simulink model "heat_exchanger_conditioning"  (R2020a)
settings: Solver=VariableStepAuto  StartTime=0.0  StopTime=1.0  RelTol=1e-3
settings Model: Creator=Mertcan  LastModifiedBy=Mertcan

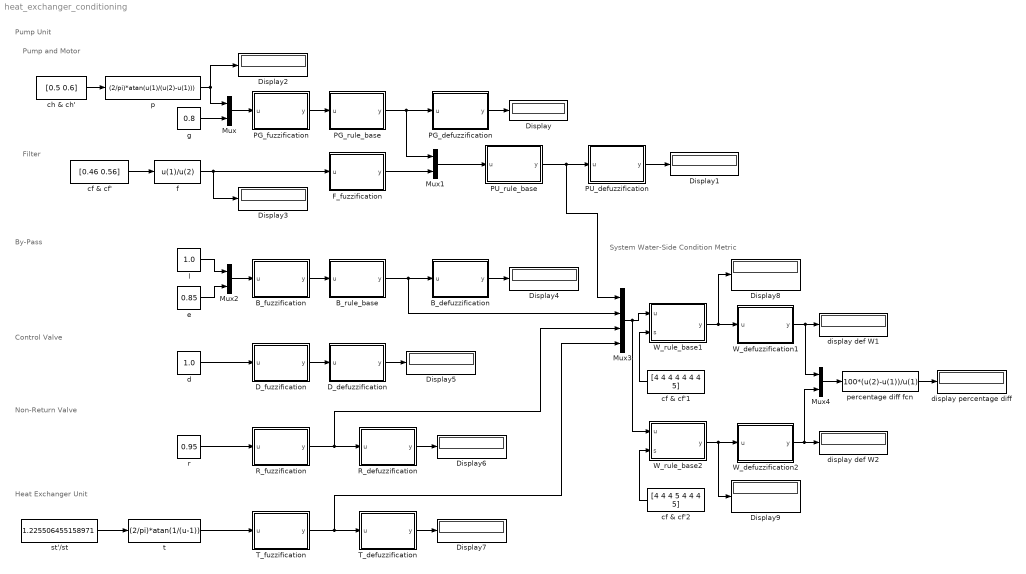
== system heat_exchanger_conditioning ==
  note: System Water-Side Condition Metric
  note: Filter
  note: Pump and Motor
  note: Heat Exchanger Unit
  note: Non-Return Valve
  note: Control Valve
  note: By-Pass
  note: Pump Unit
  B_defuzzification : MATLAB Function  TreatAsAtomicUnit=on
  B_fuzzification : MATLAB Function  TreatAsAtomicUnit=on
  B_rule_base : MATLAB Function  TreatAsAtomicUnit=on
  D_defuzzification : MATLAB Function  TreatAsAtomicUnit=on
  D_fuzzification : MATLAB Function  TreatAsAtomicUnit=on
  Display{,1..9} (10 alike) : Display
  F_fuzzification : MATLAB Function  TreatAsAtomicUnit=on
  Mux{,1..2,4} (4 alike) : Mux  Inputs=2
  Mux3 : Mux
  PG_defuzzification : MATLAB Function  TreatAsAtomicUnit=on
  PG_fuzzification : MATLAB Function  TreatAsAtomicUnit=on
  PG_rule_base : MATLAB Function  TreatAsAtomicUnit=on
  PU_defuzzification : MATLAB Function  TreatAsAtomicUnit=on
  PU_rule_base : MATLAB Function  TreatAsAtomicUnit=on
  R_defuzzification : MATLAB Function  TreatAsAtomicUnit=on
  R_fuzzification : MATLAB Function  TreatAsAtomicUnit=on
  T_defuzzification : MATLAB Function  TreatAsAtomicUnit=on
  T_fuzzification : MATLAB Function  TreatAsAtomicUnit=on
  W_defuzzification1 : MATLAB Function  TreatAsAtomicUnit=on
  W_defuzzification2 : MATLAB Function  TreatAsAtomicUnit=on
  W_rule_base1 : MATLAB Function  TreatAsAtomicUnit=on
  W_rule_base2 : MATLAB Function  TreatAsAtomicUnit=on
  cf & cf' : Constant  Value=[0.46 0.56]
  cf & cf'1 : Constant  Value=[4 4 4 4 4 4 4 5]
  cf & cf'2 : Constant  Value=[4 4 4 5 4 4 4 5]
  ch & ch' : Constant  Value=[0.5 0.6]
  d : Constant  Value=1.0
  display def W1 : Display
  display def W2 : Display
  display percentage diff : Display
  e : Constant  Value=0.85
  f : Fcn  Expr=u(1)/u(2)
  g : Constant  Value=0.8
  l : Constant  Value=1.0
  p : Fcn  Expr=(2/pi)*atan(u(1)/(u(2)-u(1)))
  percentage diff fcn : Fcn  Expr=100*(u(2)-u(1))/u(1)
  r : Constant  Value=0.95
  st'/st : Constant  Value=1.225506455158971
  t : Fcn  Expr=(2/pi)*atan(1/(u-1))
  wires:
  p/1 -> Display2/1, Mux/1
  g/1 -> Mux/2
  Mux/1 -> PG_fuzzification/1(u)
  f/1 -> Display3/1, F_fuzzification/1(u)
  PG_fuzzification/1(y) -> PG_rule_base/1(u)
  PU_defuzzification/1(y) -> Display1/1
  ch & ch'/1 -> p/1
  cf & cf'/1 -> f/1
  e/1 -> Mux2/2
  l/1 -> Mux2/1
  Mux2/1 -> B_fuzzification/1(u)
  B_fuzzification/1(y) -> B_rule_base/1(u)
  d/1 -> D_fuzzification/1(u)
  r/1 -> R_fuzzification/1(u)
  t/1 -> T_fuzzification/1(u)
  st'/st/1 -> t/1
  PG_rule_base/1(y) -> PG_defuzzification/1(u), Mux1/1
  PG_defuzzification/1(y) -> Display/1
  Mux1/1 -> PU_rule_base/1(u)
  PU_rule_base/1(y) -> Mux3/1, PU_defuzzification/1(u)
  F_fuzzification/1(y) -> Mux1/2
  B_rule_base/1(y) -> Mux3/2, B_defuzzification/1(u)
  B_defuzzification/1(y) -> Display4/1
  D_defuzzification/1(y) -> Display5/1
  D_fuzzification/1(y) -> D_defuzzification/1(u)
  R_defuzzification/1(y) -> Display6/1
  R_fuzzification/1(y) -> Mux3/3, R_defuzzification/1(u)
  T_fuzzification/1(y) -> Mux3/4, T_defuzzification/1(u)
  T_defuzzification/1(y) -> Display7/1
  Mux3/1 -> W_rule_base2/1(u), W_rule_base1/1(u)
  cf & cf'1/1 -> W_rule_base1/2(s)
  cf & cf'2/1 -> W_rule_base2/2(s)
  W_rule_base1/1(y) -> W_defuzzification1/1(u), Display8/1
  W_rule_base2/1(y) -> W_defuzzification2/1(u), Display9/1
  W_defuzzification1/1(y) -> Mux4/1, display def W1/1
  W_defuzzification2/1(y) -> Mux4/2, display def W2/1
  Mux4/1 -> percentage diff fcn/1
  percentage diff fcn/1 -> display percentage diff/1

== matlab function heat_exchanger_conditioning/T_fuzzification ==
  data: u input; y output
function y = fcn(u)

% Heat Exchanger Unit
t = u; % pump condition

T = epud(t);

y = T;

function mu = epud(x)
    mu = zeros(1,5);
    if x < 0
        mu(1) = 1+4*x;
    elseif x < 0.25
        mu(1) = 1-4*x;
        mu(2) = 4*x;
    elseif x < 0.5
        mu(2) = 2*(1-2*x);
        mu(3) = 4*x-1;
    elseif x < 0.75
        mu(3) = 3-4*x;
        mu(4) = 2*(2*x-1);
    elseif x < 1
        mu(4) = 4*(1-x);
        mu(5) = 4*x-3;
    else
        mu(5) = 5-4*x;
    end
end

end

== matlab function heat_exchanger_conditioning/W_rule_base1 ==
  data: u input; y output; s input
function y = fcn(u,s)

% System Water-Side Condition Metric

% Pump Unit
PU = u(1,1:5);

% By-Pass
B = u(1,6:10);

% Control Valve
% D: reduced without loss

% Non-Return Valve
R = u(1,11:15);

% Heat Exchanger Unit
T = u(1,16:20);

firingPU = find(PU > 0);
firingB = find(B > 0);
firingR = find(R > 0);
firingT = find(T > 0);

outPU = zeros(1,2);
outPU(1) = PU(firingPU(1));
outPU(2) = PU(firingPU(2));

outB = zeros(1,2);
outB(1) = B(firingB(1));
outB(2) = B(firingB(2));

outR = zeros(1,2);
outR(1) = R(firingR(1));
outR(2) = R(firingR(2));

outT = zeros(1,2);
outT(1) = T(firingT(1));
outT(2) = T(firingT(2));

W = ruleW(outPU,outB,outR,outT,s);

y = W;

function W = ruleW(outPU,outB,outR,outT,subscript)
    
    maxPU = max(outPU);
    
    R4 = zeros(1,8);
    R5 = zeros(1,8);
    
    if subscript(1) == 4
        R4(1) = min([maxPU,outB(1),outR(1),outT(1)]);
    elseif subscript(1) == 5
        R5(1) = min([maxPU,outB(1),outR(1),outT(1)]);
    end
    if subscript(2) == 4
        R4(2) = min([maxPU,outB(1),outR(1),outT(2)]);
    elseif subscript(2) == 5
        R5(2) = min([maxPU,outB(1),outR(1),outT(2)]);
    end
    if subscript(3) == 4
        R4(3) = min([maxPU,outB(1),outR(2),outT(1)]);
    elseif subscript(3) == 5
        R5(3) = min([maxPU,outB(1),outR(2),outT(1)]);
    end
    if subscript(4) == 4
        R4(4) = min([maxPU,outB(1),outR(2),outT(2)]);
    elseif subscript(4) == 5
        R5(4) = min([maxPU,outB(1),outR(2),outT(2)]);
    end
    if subscript(5) == 4
        R4(5) = min([maxPU,outB(2),outR(1),outT(1)]);
    elseif subscript(5) == 5
        R5(5) = min([maxPU,outB(2),outR(1),outT(1)]);
    end
    if subscript(6) == 4
        R4(6) = min([maxPU,outB(2),outR(1),outT(2)]);
    elseif subscript(6) == 5
        R5(6) = min([maxPU,outB(2),outR(1),outT(2)]);
    end
    if subscript(7) == 4
        R4(7) = min([maxPU,outB(2),outR(2),outT(1)]);
    elseif subscript(7) == 5
        R5(7) = min([maxPU,outB(2),outR(2),outT(1)]);
    end
    if subscript(8) == 4
        R4(8) = min([maxPU,outB(2),outR(2),outT(2)]);
    elseif subscript(8) == 5
        R5(8) = min([maxPU,outB(2),outR(2),outT(2)]);
    end
    
	W = [max(R4),max(R5)];    
end


end

== matlab function heat_exchanger_conditioning/W_rule_base2 ==
  data: u input; y output; s input
function y = fcn(u,s)

% System Water-Side Condition Metric

% Pump Unit
PU = u(1,1:5);

% By-Pass
B = u(1,6:10);

% Control Valve
% D: reduced without loss

% Non-Return Valve
R = u(1,11:15);

% Heat Exchanger Unit
T = u(1,16:20);

firingPU = find(PU > 0);
firingB = find(B > 0);
firingR = find(R > 0);
firingT = find(T > 0);

outPU = zeros(1,2);
outPU(1) = PU(firingPU(1));
outPU(2) = PU(firingPU(2));

outB = zeros(1,2);
outB(1) = B(firingB(1));
outB(2) = B(firingB(2));

outR = zeros(1,2);
outR(1) = R(firingR(1));
outR(2) = R(firingR(2));

outT = zeros(1,2);
outT(1) = T(firingT(1));
outT(2) = T(firingT(2));

W = ruleW(outPU,outB,outR,outT,s);

y = W;

function W = ruleW(outPU,outB,outR,outT,subscript)
    
    maxPU = max(outPU);
    
    R4 = zeros(1,8);
    R5 = zeros(1,8);
    
    if subscript(1) == 4
        R4(1) = min([maxPU,outB(1),outR(1),outT(1)]);
    elseif subscript(1) == 5
        R5(1) = min([maxPU,outB(1),outR(1),outT(1)]);
    end
    if subscript(2) == 4
        R4(2) = min([maxPU,outB(1),outR(1),outT(2)]);
    elseif subscript(2) == 5
        R5(2) = min([maxPU,outB(1),outR(1),outT(2)]);
    end
    if subscript(3) == 4
        R4(3) = min([maxPU,outB(1),outR(2),outT(1)]);
    elseif subscript(3) == 5
        R5(3) = min([maxPU,outB(1),outR(2),outT(1)]);
    end
    if subscript(4) == 4
        R4(4) = min([maxPU,outB(1),outR(2),outT(2)]);
    elseif subscript(4) == 5
        R5(4) = min([maxPU,outB(1),outR(2),outT(2)]);
    end
    if subscript(5) == 4
        R4(5) = min([maxPU,outB(2),outR(1),outT(1)]);
    elseif subscript(5) == 5
        R5(5) = min([maxPU,outB(2),outR(1),outT(1)]);
    end
    if subscript(6) == 4
        R4(6) = min([maxPU,outB(2),outR(1),outT(2)]);
    elseif subscript(6) == 5
        R5(6) = min([maxPU,outB(2),outR(1),outT(2)]);
    end
    if subscript(7) == 4
        R4(7) = min([maxPU,outB(2),outR(2),outT(1)]);
    elseif subscript(7) == 5
        R5(7) = min([maxPU,outB(2),outR(2),outT(1)]);
    end
    if subscript(8) == 4
        R4(8) = min([maxPU,outB(2),outR(2),outT(2)]);
    elseif subscript(8) == 5
        R5(8) = min([maxPU,outB(2),outR(2),outT(2)]);
    end
    
	W = [max(R4),max(R5)];    
end


end

== matlab function heat_exchanger_conditioning/W_defuzzification1 ==
  data: u input; y output
function y = fcn(u)

W = zeros(1,5);
W(4) = u(1);
W(5) = u(2);

defW = defuzzify(W);

y = defW;

function out = defuzzify(R)

    out = (R(1)*0 + R(2)*0.25 + R(3)*0.5 + R(4)*0.75 + R(5)*1)/(sum(R));

end

end

== matlab function heat_exchanger_conditioning/W_defuzzification2 ==
  data: u input; y output
function y = fcn(u)

W = zeros(1,5);
W(4) = u(1);
W(5) = u(2);

defW = defuzzify(W);

y = defW;

function out = defuzzify(R)

    out = (R(1)*0 + R(2)*0.25 + R(3)*0.5 + R(4)*0.75 + R(5)*1)/(sum(R));

end

end

== matlab function heat_exchanger_conditioning/PG_fuzzification ==
  data: u input; y output
function y = fcn(u)

% Pump and Motor
p = u(1); % pump condition
g = u(2); % assumed pump-gland condition

% Pump and Filter Condition
P = epud(p); % filter condition
G = epud(g); % gland condition

y = [P;G];

function mu = epud(x)
    mu = zeros(1,5);
    if x < 0
        mu(1) = 1+4*x;
    elseif x < 0.25
        mu(1) = 1-4*x;
        mu(2) = 4*x;
    elseif x < 0.5
        mu(2) = 2*(1-2*x);
        mu(3) = 4*x-1;
    elseif x < 0.75
        mu(3) = 3-4*x;
        mu(4) = 2*(2*x-1);
    elseif x < 1
        mu(4) = 4*(1-x);
        mu(5) = 4*x-3;
    else
        mu(5) = 5-4*x;
    end
end

end

== matlab function heat_exchanger_conditioning/B_fuzzification ==
  data: u input; y output
function y = fcn(u)

% By-Pass
l = u(1); % observed valve gland seal condition

L = epud(l);

e = u(2); % operational ease condition

E = epud_inv(e);

y = [L,E];

function mu = epud(x)
    mu = zeros(1,5);
    if x < 0
        mu(1) = 1+4*x;
    elseif x < 0.25
        mu(1) = 1-4*x;
        mu(2) = 4*x;
    elseif x < 0.5
        mu(2) = 2*(1-2*x);
        mu(3) = 4*x-1;
    elseif x < 0.75
        mu(3) = 3-4*x;
        mu(4) = 2*(2*x-1);
    elseif x < 1
        mu(4) = 4*(1-x);
        mu(5) = 4*x-3;
    else
        mu(5) = 5-4*x;
    end
end

function mu = epud_inv(x)
    mu = zeros(1,5);
    if x < 0
        mu(5) = 1+4*x;
    elseif x < 0.25
        mu(5) = 1-4*x;
        mu(4) = 4*x;
    elseif x < 0.5
        mu(4) = 2*(1-2*x);
        mu(3) = 4*x-1;
    elseif x < 0.75
        mu(3) = 3-4*x;
        mu(2) = 2*(2*x-1);
    elseif x < 1
        mu(2) = 4*(1-x);
        mu(1) = 4*x-3;
    else
        mu(1) = 5-4*x;
    end
end

end

== matlab function heat_exchanger_conditioning/D_defuzzification ==
  data: u input; y output
function y = fcn(u)

D = u;

defD = defuzzify(D);

y = defD;

function out = defuzzify(R)

    out = (R(1)*0 + R(2)*0.25 + R(3)*0.5 + R(4)*0.75 + R(5)*1)/(sum(R));

end

end

== matlab function heat_exchanger_conditioning/R_defuzzification ==
  data: u input; y output
function y = fcn(u)

R = u;

defR = defuzzify(R);

y = defR;

function out = defuzzify(R)

    out = (R(1)*0 + R(2)*0.25 + R(3)*0.5 + R(4)*0.75 + R(5)*1)/(sum(R));

end

end

== matlab function heat_exchanger_conditioning/T_defuzzification ==
  data: u input; y output
function y = fcn(u)

T = u;

defT = defuzzify(T);

y = defT;

function out = defuzzify(R)

    out = (R(1)*0 + R(2)*0.25 + R(3)*0.5 + R(4)*0.75 + R(5)*1)/(sum(R));

end

end

== matlab function heat_exchanger_conditioning/PG_rule_base ==
  data: u input; y output
function y = fcn(u)

% Pump and Filter Condition
P = u(1,:); % filter condition
G = u(2,:); % gland condition

PG = rulePG(P,G);

y = PG;

function PG = rulePG(P,G)
    R11 = min(P(1),G(1));
    R21 = min(P(1),G(2));
    R12 = min(P(2),G(1));
    R22 = min(P(2),G(2));
    R32 = min(P(2),G(3));
    R23 = min(P(3),G(2));
    R33 = min(P(3),G(3));
    R43 = min(P(3),G(4));
    R34 = min(P(4),G(3));
    R44 = min(P(4),G(4));
    R54 = min(P(4),G(5));
    R45 = min(P(5),G(4));
    R55 = min(P(5),G(5));
    
    PG = [max([R11,R21,R12]),max([R22,R32,R23]),max([R33,R43,R34]),max([R44,R54,R45]),R55];    
end

end

== matlab function heat_exchanger_conditioning/PG_defuzzification ==
  data: u input; y output
function y = fcn(u)

PG = u;

defPG = defuzzify(PG);

y = defPG;

function out = defuzzify(R)

    out = (R(1)*0 + R(2)*0.25 + R(3)*0.5 + R(4)*0.75 + R(5)*1)/(sum(R));

end

end

== matlab function heat_exchanger_conditioning/PU_rule_base ==
  data: u input; y output
function y = fcn(u)

% Pump Unit Condition
PG = u(1:5);

% Filter Condition
F = u(6:10);

PU = rulePU(PG,F);

y = PU;

function PU = rulePU(P,U)
    R11 = min(P(1),U(1));
    R21 = min(P(1),U(2));
    R12 = min(P(2),U(1));
    R22 = min(P(2),U(2));
    R32 = min(P(2),U(3));
    R23 = min(P(3),U(2));
    R33 = min(P(3),U(3));
    R43 = min(P(3),U(4));
    R34 = min(P(4),U(3));
    R44 = min(P(4),U(4));
    R54 = min(P(4),U(5));
    R45 = min(P(5),U(4));
    R55 = min(P(5),U(5));
    
    PU = [max([R11,R21]),max([R12,R22,R32,R23]),max([R33,R43,R34]),max([R44,R54,R45]),R55];    
end

end

== matlab function heat_exchanger_conditioning/F_fuzzification ==
  data: u input; y output
function y = fcn(u)

% Filter Condition
f = u;
F = epud(f); % pump condition

y = F;

function mu = epud(x)
    mu = zeros(1,5);
    if x < 0
        mu(1) = 1+4*x;
    elseif x < 0.25
        mu(1) = 1-4*x;
        mu(2) = 4*x;
    elseif x < 0.5
        mu(2) = 2*(1-2*x);
        mu(3) = 4*x-1;
    elseif x < 0.75
        mu(3) = 3-4*x;
        mu(4) = 2*(2*x-1);
    elseif x < 1
        mu(4) = 4*(1-x);
        mu(5) = 4*x-3;
    else
        mu(5) = 5-4*x;
    end
end

end

== matlab function heat_exchanger_conditioning/B_rule_base ==
  data: u input; y output
function y = fcn(u)

L = u(1:5);

E = u(6:10);

B = ruleB(E,L);

y = B;

function B = ruleB(E,L)
    R11 = min(E(5),L(1));
    R21 = min(E(5),L(2));
    R31 = min(E(5),L(3));
    R41 = min(E(5),L(4));
    R51 = min(E(5),L(5));
    R12 = min(E(4),L(1));
    R22 = min(E(4),L(2));
    R32 = min(E(4),L(3));
    R42 = min(E(4),L(4));
    R52 = min(E(4),L(5));
    R13 = min(E(3),L(1));
    R23 = min(E(3),L(2));
    R33 = min(E(3),L(3));
    R43 = min(E(3),L(4));
    R53 = min(E(3),L(5));
    R14 = min(E(2),L(1));
    R24 = min(E(2),L(2));
    R34 = min(E(2),L(3));
    R44 = min(E(2),L(4));
    R54 = min(E(2),L(5));
    R15 = min(E(1),L(1));
    R25 = min(E(1),L(2));
    R35 = min(E(1),L(3));
    R45 = min(E(1),L(4));
    R55 = min(E(1),L(5));
    
    B = [max([R11,R21,R31,R41,R51,R12,R13,R14,R15]),max([R22,R32,R42,R52,R23,R24,R25]),max([R33,R43,R53,R34,R35]),max([R44,R54,R45]),R55];    
end

end

== matlab function heat_exchanger_conditioning/PU_defuzzification ==
  data: u input; y output
function y = fcn(u)

PU = u;

defPU = defuzzify(PU);

y = defPU;

function out = defuzzify(R)

    out = (R(1)*0 + R(2)*0.25 + R(3)*0.5 + R(4)*0.75 + R(5)*1)/(sum(R));

end

end

== matlab function heat_exchanger_conditioning/B_defuzzification ==
  data: u input; y output
function y = fcn(u)

B = u;

defB = defuzzify(B);

y = defB;

function out = defuzzify(R)

    out = (R(1)*0 + R(2)*0.25 + R(3)*0.5 + R(4)*0.75 + R(5)*1)/(sum(R));

end

end

== matlab function heat_exchanger_conditioning/D_fuzzification ==
  data: u input; y output
function y = fcn(u)

% Control Valve
d = u; % the unit condition observation

D = epud(d);

y = D;

function mu = epud(x)
    mu = zeros(1,5);
    if x < 0
        mu(1) = 1+4*x;
    elseif x < 0.25
        mu(1) = 1-4*x;
        mu(2) = 4*x;
    elseif x < 0.5
        mu(2) = 2*(1-2*x);
        mu(3) = 4*x-1;
    elseif x < 0.75
        mu(3) = 3-4*x;
        mu(4) = 2*(2*x-1);
    elseif x < 1
        mu(4) = 4*(1-x);
        mu(5) = 4*x-3;
    else
        mu(5) = 5-4*x;
    end
end

end

== matlab function heat_exchanger_conditioning/R_fuzzification ==
  data: u input; y output
function y = fcn(u)

% Non-Return Valve
r = u; % the observed condition

R = epud(r);

y = R;

function mu = epud(x)
    mu = zeros(1,5);
    if x < 0
        mu(1) = 1+4*x;
    elseif x < 0.25
        mu(1) = 1-4*x;
        mu(2) = 4*x;
    elseif x < 0.5
        mu(2) = 2*(1-2*x);
        mu(3) = 4*x-1;
    elseif x < 0.75
        mu(3) = 3-4*x;
        mu(4) = 2*(2*x-1);
    elseif x < 1
        mu(4) = 4*(1-x);
        mu(5) = 4*x-3;
    else
        mu(5) = 5-4*x;
    end
end

end
